simulink model "Traction_Control_Simulation_Test_Simple_tire"  (R2016a)
settings: Solver=ode23t  StartTime=0.0  StopTime=20  RelTol=1e-3  AbsTol=1e-3
PreLoadFcn:
  | load CarSim_FE4.mat
  | load Vehicle_information_test_0118_2017.mat
libraries: fl_lib x14, nesl_utility x12, sdl_lib x4
settings Model: Creator=Ping  LastModifiedBy=Ping
settings DataIOCC: LimitDataPoints=on
settings DebuggingCC: AllowSymbolicDim=off
settings ConfigComp: CovModelRefEnable=Off  CovSFcnEnable=off
settings SimscapeCC: SimscapeLogType=all  SimscapeLogDataHistory=10000

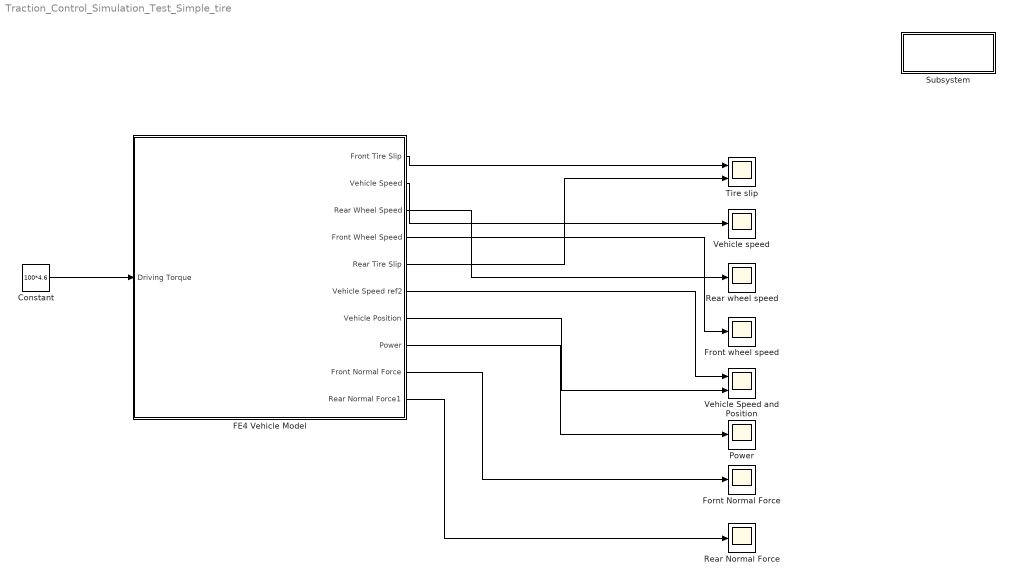
== system Traction_Control_Simulation_Test_Simple_tire ==
  Constant : Constant  Value=100*4.6
  FE4 Vehicle Model : Subsystem
  Fornt Normal Force : Scope
  Front wheel speed : Scope
  Power : Scope
  Rear Normal Force : Scope
  Rear wheel speed : Scope
  Subsystem : Subsystem
      settings: OpenFcn=open_system('simscape')
      mask Display: disp(sprintf('Open Simscape\nLibrary'));
  Tire slip : Scope  NumInputPorts=2
  Vehicle Speed and Position : Scope  NumInputPorts=2
  Vehicle speed : Scope
  wires:
  FE4 Vehicle Model/1(Front Tire Slip) -> Tire slip/1
  FE4 Vehicle Model/2(Vehicle Speed) -> Vehicle speed/1
  FE4 Vehicle Model/4(Front Wheel Speed) -> Front wheel speed/1
  Constant/1 -> FE4 Vehicle Model/1(Driving Torque)
  FE4 Vehicle Model/5(Rear Tire Slip) -> Tire slip/2
  FE4 Vehicle Model/6(Vehicle Speed ref2) -> Vehicle Speed and Position/1
  FE4 Vehicle Model/7(Vehicle Position) -> Vehicle Speed and Position/2
  FE4 Vehicle Model/3(Rear Wheel Speed) -> Rear wheel speed/1
  FE4 Vehicle Model/8(Power) -> Power/1
  FE4 Vehicle Model/9(Front Normal Force) -> Fornt Normal Force/1
  FE4 Vehicle Model/10(Rear Normal Force1) -> Rear Normal Force/1

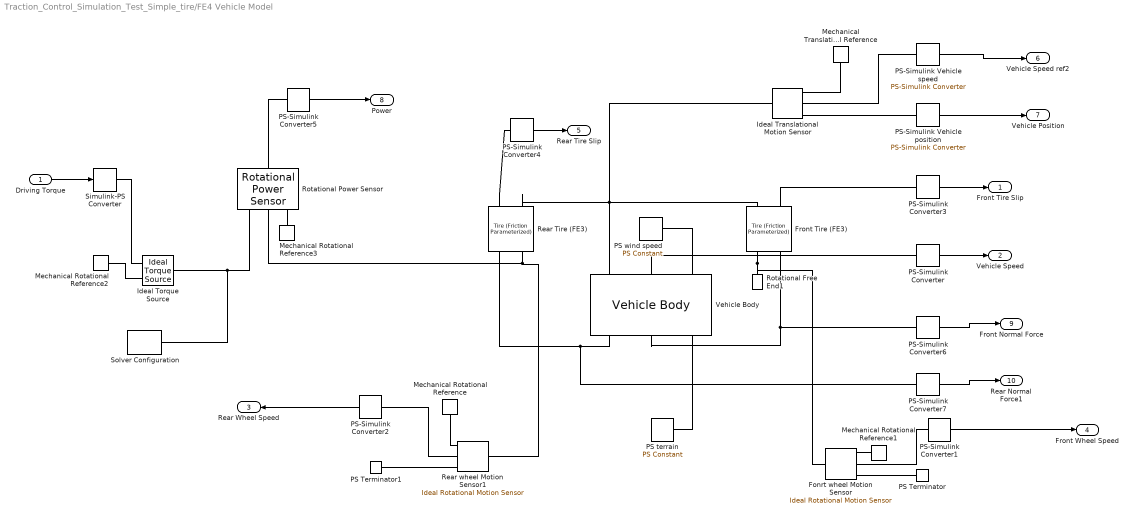
== system Traction_Control_Simulation_Test_Simple_tire/FE4 Vehicle Model ==
  Driving Torque : Inport
  Fonrt wheel Motion Sensor : fl_lib/Mechanical/Mechanical Sensors/Ideal Rotational Motion Sensor  offset=0 rad
  Front Tire (FE3) : sdl_lib/Tires & Vehicles/Tire (Friction Parameterized)  r_tire=r_tire m  mu_static=1  friction_model=1  mu_kinetic=0.7  slip_vector=SL  mu_kinetic_vector=Tire_nu  interp_method=1  extrap_method=1  model_compliance=0  stiffness=1e+6 N/m  damping=1000 N/(m/s)  model_inertia=1  tire_inertia=jt kg*m^2  initial_velocity=0 rad/s  model_resistance=0  resistance_model=1  coeff=0.015  p_tire=250e3 Pa  alpha=-0.003  beta=0.97  coeff_a=84e-4  coeff_b=6.2e-4 s/m  coeff_c=1.6e-4 s^2/m^2  v_thr=1e-3 m/s  v_tol=0.01 m/s  F_min=10 N  initial_traction_state=1
  Ideal Torque Source : fl_lib/Mechanical/Mechanical Sources/Ideal Torque Source
  Ideal Translational Motion Sensor : fl_lib/Mechanical/Mechanical Sensors/Ideal Translational Motion Sensor  offset=0 m
  Mechanical Rotational Reference{,1..3} (4 alike) : fl_lib/Mechanical/Rotational Elements/Mechanical Rotational Reference
  Mechanical Translational Reference : fl_lib/Mechanical/Translational Elements/Mechanical Translational Reference
  PS Terminator : fl_lib/Physical Signals/Sinks/PS Terminator
  PS Terminator1 : fl_lib/Physical Signals/Sinks/PS Terminator
  PS terrain : fl_lib/Physical Signals/Sources/PS Constant  constant=0
  PS wind speed : fl_lib/Physical Signals/Sources/PS Constant  constant=0
  PS-Simulink Converter : nesl_utility/PS-Simulink Converter  PhysicalDomain=network_engine_domain  SubClassName=ps_output  LeftPortType=input  RightPortType=output  PseudoPeriodic=off  Frequencies=[]  Unit=km/hr  AffineConversion=off
  PS-Simulink Converter1 : nesl_utility/PS-Simulink Converter  PhysicalDomain=network_engine_domain  SubClassName=ps_output  LeftPortType=input  RightPortType=output  PseudoPeriodic=off  Frequencies=[]  Unit=rpm  AffineConversion=off
  PS-Simulink Converter2 : nesl_utility/PS-Simulink Converter  PhysicalDomain=network_engine_domain  SubClassName=ps_output  LeftPortType=input  RightPortType=output  PseudoPeriodic=off  Frequencies=[]  Unit=rpm  AffineConversion=off
  PS-Simulink Converter3 : nesl_utility/PS-Simulink Converter  PhysicalDomain=network_engine_domain  SubClassName=ps_output  LeftPortType=input  RightPortType=output  PseudoPeriodic=off  Frequencies=[]  Unit=1  AffineConversion=off
  PS-Simulink Converter4 : nesl_utility/PS-Simulink Converter  PhysicalDomain=network_engine_domain  SubClassName=ps_output  LeftPortType=input  RightPortType=output  PseudoPeriodic=off  Frequencies=[]  Unit=1  AffineConversion=off
  PS-Simulink Converter5 : nesl_utility/PS-Simulink Converter  PhysicalDomain=network_engine_domain  SubClassName=ps_output  LeftPortType=input  RightPortType=output  PseudoPeriodic=off  Frequencies=[]  Unit=kW  AffineConversion=off
  PS-Simulink Converter6 : nesl_utility/PS-Simulink Converter  PhysicalDomain=network_engine_domain  SubClassName=ps_output  LeftPortType=input  RightPortType=output  PseudoPeriodic=off  Frequencies=[]  Unit=N  AffineConversion=off
  PS-Simulink Converter7 : nesl_utility/PS-Simulink Converter  PhysicalDomain=network_engine_domain  SubClassName=ps_output  LeftPortType=input  RightPortType=output  PseudoPeriodic=off  Frequencies=[]  Unit=N  AffineConversion=off
  PS-Simulink Vehicle position : nesl_utility/PS-Simulink Converter  PhysicalDomain=network_engine_domain  SubClassName=ps_output  LeftPortType=input  RightPortType=output  PseudoPeriodic=off  Frequencies=[]  Unit=m  AffineConversion=off
  PS-Simulink Vehicle speed : nesl_utility/PS-Simulink Converter  PhysicalDomain=network_engine_domain  SubClassName=ps_output  LeftPortType=input  RightPortType=output  PseudoPeriodic=off  Frequencies=[]  Unit=km/hr  AffineConversion=off
  Rear Tire (FE3) : sdl_lib/Tires & Vehicles/Tire (Friction Parameterized)  r_tire=r_tire m  mu_static=1  friction_model=1  mu_kinetic=0.7  slip_vector=SL  mu_kinetic_vector=Tire_nu  interp_method=1  extrap_method=1  model_compliance=0  stiffness=1e+6 N/m  damping=1000 N/(m/s)  model_inertia=1  tire_inertia=jt kg*m^2  initial_velocity=0 rad/s  model_resistance=0  resistance_model=1  coeff=0.015  p_tire=250e3 Pa  alpha=-0.003  beta=0.97  coeff_a=84e-4  coeff_b=6.2e-4 s/m  coeff_c=1.6e-4 s^2/m^2  v_thr=1e-3 m/s  v_tol=0.01 m/s  F_min=10 N  initial_traction_state=1
  Rear wheel Motion Sensor1 : fl_lib/Mechanical/Mechanical Sensors/Ideal Rotational Motion Sensor  offset=0 rad
  Rotational Free End1 : fl_lib/Mechanical/Rotational Elements/Rotational Free End  w_specify=off  w_priority=None  w=0 rad/s
  Rotational Power Sensor : sdl_lib/Sensors/Rotational Power Sensor  measurement_type=1  averaging_period=1 s  max_speed=1000 rpm  max_frequency=1000 Hz
  Simulink-PS Converter : nesl_utility/Simulink-PS Converter  PhysicalDomain=network_engine_domain  SubClassName=ps_input  LeftPortType=input  RightPortType=output  PseudoPeriodic=off  Frequencies=[]  NoiseDistribution=none  NoiseParameters=[]  Unit=N*m  AffineConversion=off  InputFiltering=off  SimscapeFilterOrder=1  InputFilterTimeConstant=0.001  UdotUserProvided=1
  Solver Configuration : nesl_utility/Solver Configuration  PhysicalDomain=network_engine_domain  SubClassName=solver  LeftPortType=input  RightPortType=generic  Accelerate=off  Tones=[]  Harmonics=[]  SimulateNoise=off  Profile=off  UseLocalSampling=off  EnableSwitchedLinearOptims=on  FrequencyDomain=off  UseCCode=off  RelTol=0.001  AbsTol=1e-06  MinStep=1e-09  ToWorkspace=off  RevertToSquareIcSolve=off  NumHomotopyIterations=100  PhasorMode=off  PhasorModeNumHarmonics=1  OverrideAbsTol=off  DoDC=off  ResidualTolerance=1e-09  UseLocalSolver=off  LocalSolverChoice=NE_BACKWARD_EULER_ADVANCER  LocalSolverSampleTime=0.001  DoFixedCost=off  MaxNonlinIter=3  MaxModeIter=2  LinearAlgebra=Sparse  DelaysMemoryBudget=1024  AutomaticFiltering=on  FilteringTimeConstant=0.001
  Vehicle Body : sdl_lib/Tires & Vehicles/Vehicle Body  mass=m_total kg  n_w=2  x_f=aa m  x_r=bb m  y_c=hf m  area=frontal_area m^2  Cd=Cd  v0=0 m/s
  Front Tire Slip : Outport
  Vehicle Speed : Outport  Port=2
  Rear Wheel Speed : Outport  Port=3
  Front Wheel Speed : Outport  Port=4
  Rear Tire Slip : Outport  Port=5
  Vehicle Speed ref2 : Outport  Port=6
  Vehicle Position : Outport  Port=7
  Power : Outport  Port=8
  Front Normal Force : Outport  Port=9
  Rear Normal Force1 : Outport  Port=10
  wires:
  PS-Simulink Converter/1 -> Vehicle Speed/1
  PS-Simulink Converter4/1 -> Rear Tire Slip/1
  PS-Simulink Vehicle speed/1 -> Vehicle Speed ref2/1
  PS-Simulink Vehicle position/1 -> Vehicle Position/1
  PS-Simulink Converter1/1 -> Front Wheel Speed/1
  PS-Simulink Converter3/1 -> Front Tire Slip/1
  PS-Simulink Converter2/1 -> Rear Wheel Speed/1
  Driving Torque/1 -> Simulink-PS Converter/1
  PS-Simulink Converter5/1 -> Power/1
  PS-Simulink Converter6/1 -> Front Normal Force/1
  PS-Simulink Converter7/1 -> Rear Normal Force1/1
  connections:
  Rear Tire (FE3)/RConn2 -- Front Tire (FE3)/RConn2 -- Ideal Translational Motion Sensor/LConn1 -- Vehicle Body/LConn1
  Vehicle Body/RConn2 -- Front Tire (FE3)/LConn1 -- PS-Simulink Converter6/LConn1
  Vehicle Body/LConn2 -- PS-Simulink Converter/LConn1
  Vehicle Body/RConn1 -- PS-Simulink Converter7/LConn1 -- Rear Tire (FE3)/LConn1
  Rear wheel Motion Sensor1/RConn2 -- PS-Simulink Converter2/LConn1
  Ideal Translational Motion Sensor/RConn3 -- PS-Simulink Vehicle position/LConn1
  PS Terminator1/LConn1 -- Rear wheel Motion Sensor1/RConn3
  Ideal Translational Motion Sensor/RConn1 -- Mechanical Translational Reference/LConn1
  Fonrt wheel Motion Sensor/LConn1 -- Rotational Free End1/LConn1 -- Front Tire (FE3)/LConn2
  Front Tire (FE3)/RConn1 -- PS-Simulink Converter3/LConn1
  Rear wheel Motion Sensor1/LConn1 -- Rotational Power Sensor/LConn2 -- Rear Tire (FE3)/LConn2
  Mechanical Rotational Reference1/LConn1 -- Fonrt wheel Motion Sensor/RConn1
  Ideal Translational Motion Sensor/RConn2 -- PS-Simulink Vehicle speed/LConn1
  PS terrain/RConn1 -- Vehicle Body/RConn3
  Fonrt wheel Motion Sensor/RConn2 -- PS-Simulink Converter1/LConn1
  PS wind speed/RConn1 -- Vehicle Body/LConn3
  Rear Tire (FE3)/RConn1 -- PS-Simulink Converter4/LConn1
  PS Terminator/LConn1 -- Fonrt wheel Motion Sensor/RConn3
  Mechanical Rotational Reference/LConn1 -- Rear wheel Motion Sensor1/RConn1
  Simulink-PS Converter/RConn1 -- Ideal Torque Source/RConn1
  Mechanical Rotational Reference2/LConn1 -- Ideal Torque Source/RConn2
  Mechanical Rotational Reference3/LConn1 -- Rotational Power Sensor/LConn3
  PS-Simulink Converter5/LConn1 -- Rotational Power Sensor/RConn1
  Ideal Torque Source/LConn1 -- Solver Configuration/RConn1 -- Rotational Power Sensor/LConn1

== system Traction_Control_Simulation_Test_Simple_tire/Subsystem ==
